simulink model "state_space_try"  (R2016b)
settings: Solver=VariableStepAuto  StartTime=0.0  StopTime=100  RelTol=1e-3  EnableMultiTasking=on
values from neighbouring files (symbols this model uses):
  Ad = 0.606534330298    [sysd.mat]    (also in trock.m = sysd.A)
  Bd = [0.174938920468 0.0949331738452]    [sysd.mat]    (also in trock.m = [ sysd.B(5) sysd.B(6) ])
  Cd = [-0.336235271119 -0.0680877309367]    [sysd.mat]    (also in trock.m = [ sysd.C(2); sysd.C(4) ])
  Dd = [-0.828379120281  -0.766604322843; 0.839705991402  -0.601474126995]    [sysd.mat]    (also in trock.m = [ sysd.D(2,5) sysd.D(2,6); sysd.D(4,5) sysd.D(4,6) ])
  Ed = [ sysd.B(2) sysd.B(4)]    [trock.m]
  Kd = [ sysd.D(2,2) sysd.D(2,4); sysd.D(4,2) sysd.D(4,4) ]    [trock.m]
  Ts = 6.4385    [sysd.mat]    (also in trock.m)
libraries: powerlib_meascontrol x4
settings Model: Creator=Trojass  LastModifiedBy=CBalla
settings OptimizationCC: LifeSpan=inf
settings DebuggingCC: SFUnexpectedBacktrackingDiag=warning  SFNoUnconditionalDefaultTransitionDiag=warning  SFExecutionAtInitializationDiag=none
settings GRTTargetCC: TargetLangStandard=C89/C90 (ANSI)  GeneratePreprocessorConditionals=Disable all
settings ConfigComp: CovMetricSettings=dw  CovHtmlReporting=on  CovSaveCumulativeToWorkspaceVar=on  CovSaveSingleToWorkspaceVar=on  CovExternalEMLEnable=off

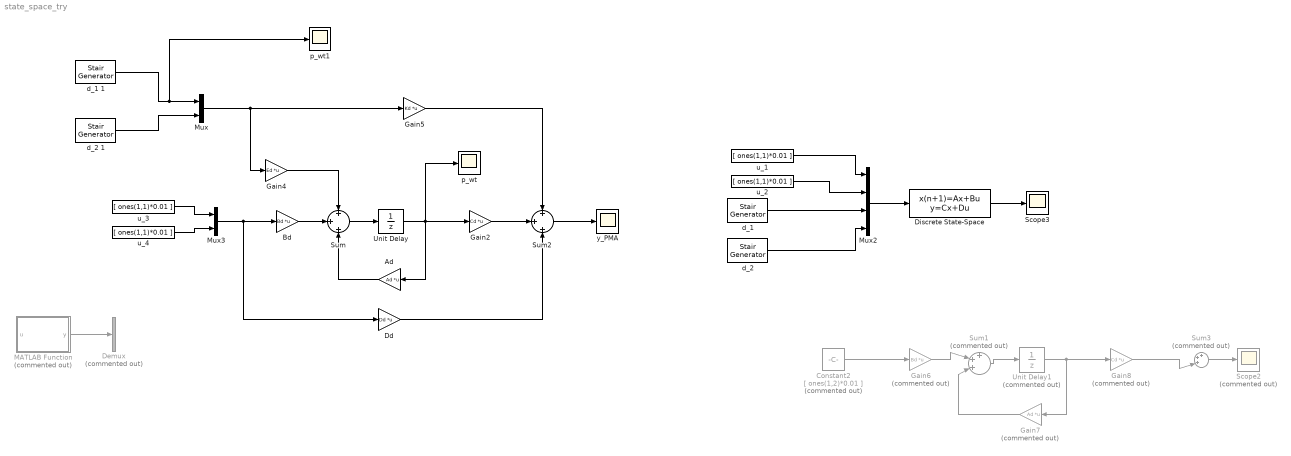
== system state_space_try ==
  Ad : Gain  Gain=Ad  Multiplication=Matrix(K*u)
      mask Display:
      | %color('cyan')
      | color('magenta')
      | disp('{\bf\fontsize{14}Ad}', 'texmode','on');
      | %disp('Ad')
  Bd : Gain  Gain=Bd  Multiplication=Matrix(K*u)
      mask Display:
      | %color('cyan')
      | color('magenta')
      | disp('{\bf\fontsize{14}Bd}', 'texmode','on');
      | %disp('Bd')
  Constant2 : Constant  Commented=on  Value=[ ones(1,2)*0.01 ]  SampleTime=Ts
  Dd : Gain  Gain=Dd  Multiplication=Matrix(K*u)
      mask Display:
      | %color('cyan')
      | color('magenta')
      | disp('{\bf\fontsize{14}Dd}', 'texmode','on');
      | %disp('Dd')
  Demux : Demux  Commented=on  Outputs=2
  Discrete State-Space : DiscreteStateSpace  A=Ad  B=[Bd Ed]  C=Cd  D=[Dd Kd]  SampleTime=Ts
  Gain2 : Gain  Gain=Cd  Multiplication=Matrix(K*u)
      mask Display:
      | %color('cyan')
      | color('magenta')
      | disp('{\bf\fontsize{14}Cd}', 'texmode','on');
      | %disp('Cd')
  Gain4 : Gain  Gain=Ed  Multiplication=Matrix(K*u)
      mask Display:
      | %color('cyan')
      | color('magenta')
      | disp('{\bf\fontsize{14}Ed}', 'texmode','on');
      | %disp('Ed')
  Gain5 : Gain  Gain=Kd  Multiplication=Matrix(K*u)
      mask Display:
      | %color('cyan')
      | color('magenta')
      | disp('{\bf\fontsize{14}Kd}', 'texmode','on');
      | %disp('Kd')
  Gain6 : Gain  Commented=on  Gain=Bd  Multiplication=Matrix(K*u)
  Gain7 : Gain  Commented=on  Gain=Ad  Multiplication=Matrix(K*u)
  Gain8 : Gain  Commented=on  Gain=Cd  Multiplication=Matrix(K*u)
  MATLAB Function : MATLAB Function  Commented=on  TreatAsAtomicUnit=on
  Mux : Mux  Inputs=2
  Mux2 : Mux
  Mux3 : Mux  Inputs=2
  Scope2 : Scope  Commented=on
  Scope3 : Scope
  Sum : Sum  Inputs=+|+|+
  Sum1 : Sum  Commented=on  Inputs=+++|
  Sum2 : Sum  Inputs=+|+|+
  Sum3 : Sum  Commented=on  Inputs=+++|
  Unit Delay : UnitDelay  SampleTime=Ts
  Unit Delay1 : UnitDelay  Commented=on  SampleTime=Ts
  "d_1 " : powerlib_meascontrol/Pulse & Signal Generators/Stair Generator  t=t  e=Data_OD  Ts=Ts
  d_1 1 : powerlib_meascontrol/Pulse & Signal Generators/Stair Generator  t=t  e=Data_OD  Ts=Ts
  "d_2 " : powerlib_meascontrol/Pulse & Signal Generators/Stair Generator  t=t  e=Data_OD  Ts=Ts
  d_2 1 : powerlib_meascontrol/Pulse & Signal Generators/Stair Generator  t=t  e=Data_OD  Ts=Ts
  p_wt : Scope
  p_wt1 : Scope
  u_{1..4} (4 alike) : Constant  Value=[ ones(1,1)*0.01 ]  SampleTime=Ts
  y_PMA : Scope
  wires:
  Sum/1 -> Unit Delay/1
  Unit Delay/1 -> p_wt/1, Gain2/1, Ad/1
  Mux3/1 -> Dd/1, Bd/1
  Bd/1 -> Sum/2
  Ad/1 -> Sum/3
  Sum2/1 -> y_PMA/1
  Gain5/1 -> Sum2/1
  Gain4/1 -> Sum/1
  Mux/1 -> Gain4/1, Gain5/1
  Sum1/1 -> Unit Delay1/1
  Unit Delay1/1 -> Gain8/1, Gain7/1
  Constant2/1 -> Gain6/1
  Gain6/1 -> Sum1/2
  Gain7/1 -> Sum1/3
  Gain8/1 -> Sum3/3
  Sum3/1 -> Scope2/1
  Discrete State-Space/1 -> Scope3/1
  Mux2/1 -> Discrete State-Space/1
  u_1/1 -> Mux2/1
  u_2/1 -> Mux2/2
  "d_1 "/1 -> Mux2/3
  "d_2 "/1 -> Mux2/4
  MATLAB Function/1(y) -> Demux/1
  d_1 1/1 -> p_wt1/1, Mux/1
  d_2 1/1 -> Mux/2
  Gain2/1 -> Sum2/2
  Dd/1 -> Sum2/3
  u_3/1 -> Mux3/1
  u_4/1 -> Mux3/2

== matlab function state_space_try/MATLAB Function ==
  data: u input; y output
function y = fcn(u)

Matrix_op;
trock;                  %Load system matrices
delta_p_0 = u;      %small-signal initial WT pressure measurement

d_hp = 0.05*90*ones(48,1);      % Small signal deviation of the Valves OD
U_bar_hp = 0.2*ones(48,1);      % Input pressure to ring pumps operating point
q_bar_p_hp = 1.4*ones(48,1);    % Flow operating point of the ring pumps

% Output constraint
y_low =  0.08*ones(48,1);         % Full-signal upper and lower bounds 
y_high = 0.18*ones(48,1);           

% Pressure operating point of the PMA end-users
y_bar = [0.1562; 0.0991 ;0.1562; 0.0991 ;0.1562; 0.0991 ;0.1562; 0.0991 ;0.1562; 0.0991 ;0.1562; 0.0991 ;
        0.1562; 0.0991 ;0.1562; 0.0991 ;0.1562; 0.0991 ;0.1562; 0.0991 ;0.1562; 0.0991 ;0.1562; 0.0991 ;
        0.1562; 0.0991 ;0.1562; 0.0991 ;0.1562; 0.0991 ;0.1562; 0.0991 ;0.1562; 0.0991 ;0.1562; 0.0991 ;
        0.1562; 0.0991 ;0.1562; 0.0991 ;0.1562; 0.0991 ;0.1562; 0.0991 ;0.1562; 0.0991 ;0.1562; 0.0991];    

y1 = y_low - y_bar - Theta*Phi*delta_p_0-(Theta*Psi+Pi)*d_hp;
y2 = y_high - y_bar - Theta*Phi*delta_p_0-(Theta*Psi+Pi)*d_hp;
L_y = Theta*Gamma+Omega;

% State constraint
x_low = 0.055*ones(24,1);
x_high = 0.164*ones(24,1);
x_bar = 0.127*ones(24,1);

delta_p_wt_1 = x_low-x_bar - Phi*delta_p_0 - Psi*d_hp;
delta_p_wt_2 = x_high-x_bar - Phi*delta_p_0 - Psi*d_hp;

% input constraint 
u_low = -0.2;
u_high = 1;

%%%%%%%%%%%%%%%%%%%%%%%%%%%%%%%%%%%%%%%%%%%%%%%%%%%%%%%
%%%%%%%%%%%%%%%%%% Setting up the QP %%%%%%%%%%%%%%%%%% 
%%%%%%%%%%%%%%%%%%%%%%%%%%%%%%%%%%%%%%%%%%%%%%%%%%%%%%%

R = 2*(Lambda_A + Lambda_C*Gamma); 
R1=(R+R')/2;
R2=(R-R')/2;
f = U_bar_hp'*(Lambda_A+Lambda_C*Gamma)+d_hp'*(Lambda_B+Lambda_C*Psi)'+delta_p_0*(Lambda_C*Phi)'+q_bar_p_hp';

%CONSTRAINTS FOR Y AND X
A = [-L_y; L_y; -Gamma; Gamma];
b = [y1; y2; delta_p_wt_1; delta_p_wt_2];

%CONSTRAINTS only FOR Y
% A = [-L_y; L_y];
% b = [y1; y2];

%CONSTRAINTS only FOR X
% A = [-Gamma;Gamma];
% b = [delta_p_wt_1; delta_p_wt_2];

lb = u_low*ones(48,1);
ub = u_high*ones(48,1);

options = optimoptions('quadprog','Algorithm','interior-point-convex','Display','iter-detailed')
[u_hp,fval,exitflag,output,lambda] = quadprog(R1,f,[],[],[],[],lb,ub,[],options);


y = [u_hp(1) u_hp(2)];
